simulink model "InvPen_Model_OpenLoop"  (R2024b)
settings: Solver=VariableStepAuto  StartTime=0.0  StopTime=9.0  RelTol=1e-3
values from neighbouring files (symbols this model uses):
  b = 0.1    [InvPen_Values.m]
  g = 9.8    [InvPen_Values.m]
  I = 0.006    [InvPen_Values.m]
  l = 0.3    [InvPen_Values.m]
  m = 0.2    [InvPen_Values.m]
  M = 0.5    [InvPen_Values.m]
settings Model: Creator=Arghya  LastModifiedBy=Arghya

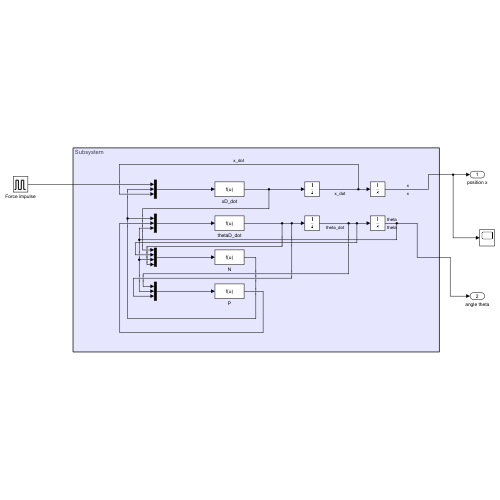
[thumbnail: Simulink's stored preview of the top-level diagram]
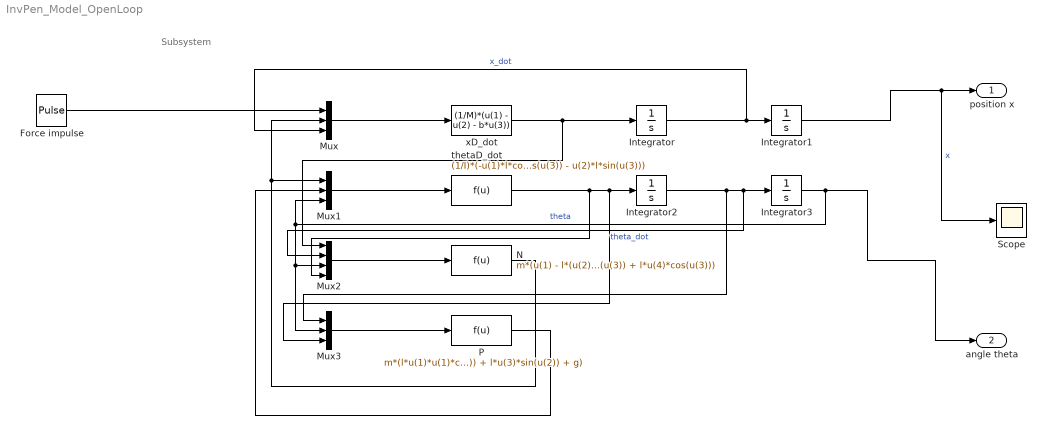
== system InvPen_Model_OpenLoop ==
  note: Subsystem
  Force impulse : DiscretePulseGenerator  PulseType=Time based  Period=10  PulseWidth=5
  Integrator : Integrator  ContinuousStateAttributes="\"x_dot\""
  Integrator1 : Integrator  ContinuousStateAttributes="\"x\""
  Integrator2 : Integrator  ContinuousStateAttributes="\"theta_dot\""
  Integrator3 : Integrator  InitialCondition=pi  ContinuousStateAttributes="\"theta\""
  Mux : Mux  Inputs=3
  Mux1 : Mux  Inputs=3
  Mux2 : Mux
  Mux3 : Mux  Inputs=3
  N : Fcn  Expr=m*(u(1) - l*(u(2)^2)*sin(u(3)) + l*u(4)*cos(u(3)))
  P : Fcn  Expr=m*(l*u(1)*u(1)*cos(u(2)) + l*u(3)*sin(u(2)) + g)
  Scope : Scope
  thetaD_dot : Fcn  Expr=(1/I)*(-u(1)*l*cos(u(3)) - u(2)*l*sin(u(3)))
  xD_dot : Fcn  Expr=(1/M)*(u(1) - u(2) - b*u(3))
  position x : Outport
  angle theta : Outport  Port=2
  wires:
  Integrator1/1 -> Scope/1, position x/1  "x"
  Mux2/1 -> N/1
  thetaD_dot/1 -> Mux2/4, Mux3/3, Integrator2/1
  Mux1/1 -> thetaD_dot/1
  P/1 -> Mux1/2
  Mux/1 -> xD_dot/1
  N/1 -> Mux1/1, Mux/2
  Integrator/1 -> Mux/3, Integrator1/1  "x_dot"
  Integrator2/1 -> Mux3/1, Mux2/2, Integrator3/1  "theta_dot"
  Integrator3/1 -> Mux3/2, Mux2/3, Mux1/3, angle theta/1  "theta"
  xD_dot/1 -> Mux2/1, Integrator/1
  Mux3/1 -> P/1
  Force impulse/1 -> Mux/1
